simulink model "UARTReadLine - Kopie"  (R2017b)
settings: Solver=FixedStepDiscrete  StartTime=0.0  StopTime=10.0  FixedStep=1e-3  RelTol=1e-3
libraries: mbed_lib x5
settings Model: Creator=oh  LastModifiedBy=oh
settings DataIOCC: LimitDataPoints=on  SaveFormat=Array
settings OptimizationCC: LifeSpan=1
settings DebuggingCC: SFUnexpectedBacktrackingDiag=warning  SFNoUnconditionalDefaultTransitionDiag=warning  SFExecutionAtInitializationDiag=none
settings HardwareCC: ProdBitPerPointer=32  ProdBitPerSizeT=32  ProdBitPerPtrDiffT=32  ProdLargestAtomicInteger=Long  ProdLargestAtomicFloat=Double  ProdIntDivRoundTo=Undefined  ProdWordSize=32  ProdHWDeviceType=ARM Compatible->ARM Cortex
settings ModelReferenceCC: PropagateSignalLabelsOutOfModel=off
settings SFSimCC: MATLABDynamicMemAlloc=off
settings RTWCC: SystemTargetFile=mbed.tlc  TemplateMakefile=mbed.tmf  Description=Mbed Target (Embedded Target)  TargetLang=C++
settings CodeAppCC: IgnoreCustomStorageClasses=off  StateflowObjectComments=on
settings STFCustomTargetCC: TargetLibSuffix=.a  GenerateSampleERTMain=on  CombineOutputUpdateFcns=on  ERTCustomFileBanners=on  SupportContinuousTime=off  SupportNonInlinedSFcns=off  RemoveResetFunc=on  SupportVariableSizeSignals=on  MATLABClassNameForMDSCustomization=Simulink.SoftwareTarget.ERTCustomization  ModelStepFunctionPrototypeControlCompliant=on  GRTInterface=off  SystemTargetFile=mbed.tlc
settings ERTTargetCC: MultiwordLength=2048  GenerateSampleERTMain=on  ParMdlRefBuildCompliant=off  CompOptLevelCompliant=off  ConcurrentExecutionCompliant=off  SupportVariableSizeSignals=on  CPPClassGenCompliant=off  UseToolchainInfoCompliant=off  ERTCustomFileTemplate=mbed_file_process.tlc  ConvertIfToSwitch=off  SuppressUnreachableDefaultCases=off
settings ConfigComp: CovMetricSettings=dw  CovHtmlReporting=on  CovSaveCumulativeToWorkspaceVar=on  CovSaveSingleToWorkspaceVar=on  CovExternalEMLEnable=off

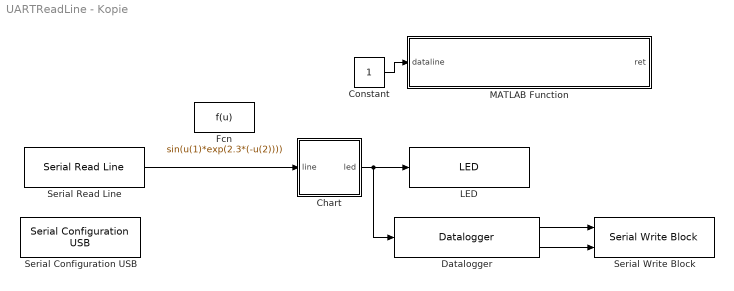
== system UARTReadLine - Kopie ==
  Chart : Stateflow chart  TreatAsAtomicUnit=on
  Constant : Constant
  Datalogger : mbed_lib/Utilities/Datalogger  TypeInputPorts={ 'uint8' 1 }  TypeOfInputs={'1*uint8'}  BufferSize=4  errEn=off  SampleTime=-1
      settings: SourceProductName=Mbed Target
  Fcn : Fcn  Expr=sin(u(1)*exp(2.3*(-u(2))))
  LED : mbed_lib/GPIO/LED  nLED=1  SampleTime=-1
      settings: SourceProductName=Mbed Target
  MATLAB Function : MATLAB Function  TreatAsAtomicUnit=on
  Serial Configuration USB : mbed_lib/Serial/UART/Serial Configuration USB  Priority=0  BaudRate=9600
      settings: AttributesFormatString=%<Priority>=10  SourceProductName=Mbed Target
  Serial Read Line : mbed_lib/Serial/UART/Serial Read Line  SerialPort=USB  numData=off  Blocking=on  BufferSize=5  SampleTime=0.5
      settings: SourceProductName=Mbed Target
  Serial Write Block : mbed_lib/Serial/UART/Serial Write Block  SerialPort=USB  numData=on  SampleTime=-1
      settings: SourceProductName=Mbed Target
  wires:
  Serial Read Line/1 -> Chart/1(line)
  Chart/1(led) -> Datalogger/1, LED/1
  Datalogger/1 -> Serial Write Block/1
  Datalogger/2 -> Serial Write Block/2
  Constant/1 -> MATLAB Function/1(dataline)

== matlab function UARTReadLine - Kopie/MATLAB Function ==
  data: ret output; dataline input
function ret = strmulticompare(dataline)

commands = {'on', 'off'};
ret = uint8(0);

for i=1:size(commands,2)
    ok=uint8(1);
    for j=1:size(commands{i},2)
        if commands{i}(j)~=dataline(j)
            ok=uint8(0);
            break;
        end
    end
    if ok==uint8(1)
      ret = uint8(i);
      return;
    end
end

== stateflow chart UARTReadLine - Kopie/Chart ==
  state on
  state start
  state off
  (default) -> start
  start -> on [order 1] : [strmulticompare({'on', 'off'}, line)==uint8(1)]
  on -> start : {led=1;}
  off -> start : {led=0;}
  start -> off [order 2] : [strmulticompare({'on', 'off'}, line)==uint8(2)]
  data: commands function_input; dataline function_input; ret function_output; line input; led output uint8
  function ret = strmulticompare(commands, dataline):
    | function ret = strmulticompare(commands, dataline)
    | 
    | %commands = {'on', 'off'};
    | ret = uint8(0);
    | 
    | for i=1:size(commands,2)
    |     ok=uint8(1);
    |     for j=1:size(commands{i},2)
    |         if commands{i}(j)~=dataline(j)
    |             ok=uint8(0);
    |             break;
    |         end
    |     end
    |     if ok==uint8(1)
    |       ret = uint8(i);
    |       return;
    |     end
    | end
